simulink model "iso_calc_temp_ver3"  (R2020a)
settings: Solver=VariableStepAuto  StartTime=0.0  StopTime=inf  RelTol=1e-6
values from neighbouring files (symbols this model uses):
  C = 1    [DataLoop.m]    (also in run_iso_calc.m; testLoop.m = 1.2)
  t_current = 0    [DataLoop.m]    (also in run_iso_calc.m = (0:t_process:tf)'; testLoop.m)
  Tr = 1    [DataLoop.m]    (also in run_iso_calc.m = 0; testLoop.m = 0.38)
  Ts = 1    [DataLoop.m]    (also in run_iso_calc.m = 0; testLoop.m = 0.5)
  Vs = 1    [DataLoop.m]    (also in run_iso_calc.m = -Vh; testLoop.m = 0)
  Zd = 1    [DataLoop.m]    (also in run_iso_calc.m = 0.05; testLoop.m = 0.02)
  Zr = 1    [DataLoop.m]    (also in run_iso_calc.m = 0; testLoop.m = 0)
libraries: simulink x1
settings Model: Creator=laiy

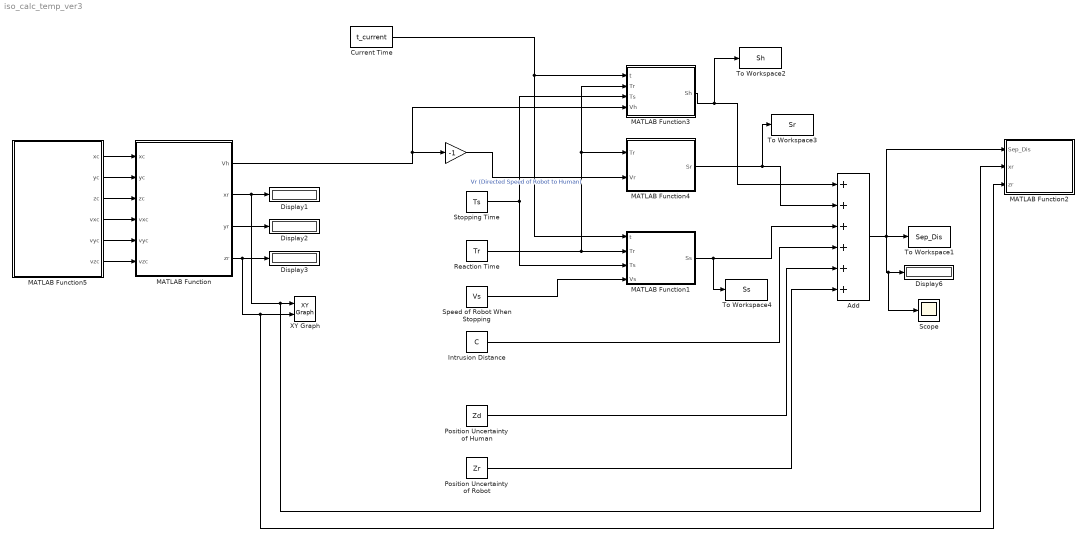
== system iso_calc_temp_ver3 ==
  " " : Gain  Gain=-1
  Add : Sum  Inputs=++++++
  Current Time : Constant  Value=t_current
  Display{1..3,6} (4 alike) : Display
  Intrusion Distance : Constant  Value=C
  MATLAB Function : MATLAB Function  TreatAsAtomicUnit=on
  MATLAB Function1 : MATLAB Function  TreatAsAtomicUnit=on
  MATLAB Function2 : MATLAB Function  TreatAsAtomicUnit=on
  MATLAB Function3 : MATLAB Function  TreatAsAtomicUnit=on
  MATLAB Function4 : MATLAB Function  TreatAsAtomicUnit=on
  MATLAB Function5 : MATLAB Function  TreatAsAtomicUnit=on
  Position Uncertainty of Human : Constant  Value=Zd
  Position Uncertainty of Robot : Constant  Value=Zr
  Reaction Time : Constant  Value=Tr
  Scope : Scope
  Speed of Robot When Stopping : Constant  Value=Vs
  Stopping Time : Constant  Value=Ts
  To Workspace1 : ToWorkspace  VariableName=Sep_Dis  SampleTime=-1
  To Workspace2 : ToWorkspace  VariableName=Sh  SampleTime=-1
  To Workspace3 : ToWorkspace  VariableName=Sr  SampleTime=-1
  To Workspace4 : ToWorkspace  VariableName=Ss  SampleTime=-1
  XY Graph : simulink/Sinks/XY Graph  xmin=-10  xmax=10  ymin=10  ymax=10  st=-1
  wires:
  MATLAB Function1/1(Ss) -> To Workspace4/1, Add/3
  MATLAB Function3/1(Sh) -> To Workspace2/1, Add/1
  MATLAB Function4/1(Sr) -> To Workspace3/1, Add/2
  Intrusion Distance/1 -> Add/4
  Position Uncertainty of Human/1 -> Add/5
  Position Uncertainty of Robot/1 -> Add/6
  Reaction Time/1 -> MATLAB Function1/2(Tr), MATLAB Function4/1(Tr), MATLAB Function3/2(Tr)
  Stopping Time/1 -> MATLAB Function3/3(Ts), MATLAB Function1/3(Ts)
  " "/1 -> MATLAB Function4/2(Vr)  "Vr (Directed Speed of Robot to Human)"
  Current Time/1 -> MATLAB Function1/1(t), MATLAB Function3/1(t)
  Speed of Robot When Stopping/1 -> MATLAB Function1/4(Vs)
  Add/1 -> MATLAB Function2/1(Sep_Dis), Scope/1, Display6/1, To Workspace1/1
  MATLAB Function/1(Vh) -> MATLAB Function3/4(Vh), " "/1
  MATLAB Function/2(xr) -> MATLAB Function2/2(xr), XY Graph/1, Display1/1
  MATLAB Function/3(yr) -> Display2/1
  MATLAB Function5/1(xc) -> MATLAB Function/1(xc)
  MATLAB Function5/2(yc) -> MATLAB Function/2(yc)
  MATLAB Function5/3(zc) -> MATLAB Function/3(zc)
  MATLAB Function5/4(vxc) -> MATLAB Function/4(vxc)
  MATLAB Function5/5(vyc) -> MATLAB Function/5(vyc)
  MATLAB Function5/6(vzc) -> MATLAB Function/6(vzc)
  MATLAB Function/4(zr) -> XY Graph/2, MATLAB Function2/3(zr), Display3/1

== matlab function iso_calc_temp_ver3/MATLAB Function4 ==
  data: Tr input; Vr input; Sr output
function Sr = fcn(Tr, Vr)

% separation distance due to robot motion
% Vr is assumed to reduces the separation distance the most

Sr = Tr * Vr;

== matlab function iso_calc_temp_ver3/MATLAB Function3 ==
  data: t input; Sh output; Tr input; Ts input; Vh input
function Sh = fcn(t, Tr, Ts, Vh)

% separation distance due to operator's change in location

t_int = t:0.001:t+Tr+Ts;
v = zeros(length(t_int),1) + Vh;

Sh = trapz(t_int,v);

== matlab function iso_calc_temp_ver3/MATLAB Function1 ==
  data: t input; Tr input; Ss output; Ts input; Vs input
function Ss = fcn(t, Tr, Ts, Vs)

% separation distance due to robot stopping

t_int = t+Tr:0.001:t+Tr+Ts;
v = zeros(length(t_int),1) + Vs;

Ss = trapz(t_int,v);

== matlab function iso_calc_temp_ver3/MATLAB Function2 ==
  data: Sep_Dis input; xr input; zr input
function display(Sep_Dis, xr,zr)

fprintf(1, 'Separation Distance: %f\n', Sep_Dis(1,1));

fileID = fopen('output.txt','w');
fprintf(fileID,'%f\n',Sep_Dis);
fclose(fileID);


f = figure(1);
title('Separation Distance');
plot(xr*5,zr*5,'o','MarkerSize', 3, 'MarkerFaceColor', 'black');
hold on;
plot(0,0,'o','MarkerSize',1, 'LineWidth', 3, 'Color', 'Red','MarkerSize', int8(abs(Sep_Dis)*100));
hold off;
xlim([-5,5]);
ylim([-5,5]);

if sqrt(xr^2 + zr^2) <= Sep_Dis
    fprintf(1,'DANGER');
end

== matlab function iso_calc_temp_ver3/MATLAB Function ==
  data: xc input; Vh output; yc input; zc input; vxc input; vyc input; vzc input; xr output; yr output; zr output
function [Vh,xr,yr,zr] = find_Vh(xc,yc,zc,vxc,vyc,vzc)

[xr,yr,zr,vxr,vyr,vzr] = trans_cam_rob(xc,yc,zc,vxc,vyc,vzc);

Vh = sqrt(vxr^2 + vzr^2);

== matlab function iso_calc_temp_ver3/MATLAB Function5 ==
  data: xc output; yc output; zc output; vxc output; vyc output; vzc output
function [xc,yc,zc,vxc,vyc,vzc] =SSMdatacall()
% The function is intended to be a constant communication call between ROS2
% and Simulink.
%   This function subscribes to the nodes and writes the data into the
%   variables needed for processing by the Simulink model. Add subscriber
%   notes in the same fashion to call any more data from the
%   ROS2-data-analytics package output.

% Variables currently needed by simulink model: xc, yc, zc ,vxc, vyc, vzc
% For first run purposes, position will be max position of bounding box.
i = 0
poseLocalData = receive(localization,10)
poseMovementData = receive(movement,10)
vxc = poseMovementData.objects.velocity.x;
vyc = poseMovementData.objects.velocity.y;
vzc = poseMovementData.objects.velocity.z;
xc  = poseMovementData.objects.max.x;
yc  = poseMovementData.objects.max.y;
zc  = poseMovementData.objects.max.c;
